simulink model "sm_radial_engine"  (R2021b)
settings: Solver=ode23t  StartTime=0.0  StopTime=10  RelTol=1e-3  EnableMultiTasking=on
model workspace (MATLAB code in the model file):
  | dgrey = [0.5 0.5 0.5];
  | lgrey = [0.7 0.7 0.7];
  | orange = [205 133 63]/255;
  | brown = [0.3 0.2 0.0];
  | lbrown = [139 90 43]/255;
  | yellow = [0.9 0.7 0.2];
  | 
  | rho_alum = 2700;
  | rho_steel = 8100;
  | 
  | Patm = 101100;
undefined symbols (not defined in the file): X, Y, Z
libraries: sm_lib x50, sm_radial_engine_lib x29, nesl_utility x2
(part 1 of 2)
Description:
  | Translational Interface : Radial Engine with Gas Force Model
  | 
  | This model simulates a five cylinder radial engine. The pressure dynamics inside the cylinders are modelled using the Simscape(TM) gas library. The 3D mechanical
  | components are modelled using Simscape Multibody(TM). See inside any of the blocks called "Force Model" to see how the 1D and 3D mechanical parts of the model are
  | interfaced. The pressure model is an ideal pressure source which applies pressure based on the crank angle. This model can be replaced with a more realistic pressure model
  | of the cylinder chamber. The cylinders fire in the sequence - A C E B D providing a power stroke every 144 deg of crank rotation.
settings Model: Creator=The MathWorks, Inc.  LastModifiedBy=The MathWorks, Inc.
settings SolverCC: AlgebraicLoopSolver=TrustRegion
settings DataIOCC: LimitDataPoints=on  SaveFormat=Array  SaveOutput=off  SignalLogging=off  SaveTime=off  ReturnWorkspaceOutputs=off  Refine=4
settings OptimizationCC: ExpressionDepthLimit=2147483647  LifeSpan=inf
settings DebuggingCC: ReadBeforeWriteMsg=DisableAll  WriteAfterWriteMsg=DisableAll  WriteAfterReadMsg=DisableAll  UnderspecifiedInitializationDetection=Classic  MergeDetectMultiDrivingBlocksExec=none  StateNameClashWarn=warning  SFUnexpectedBacktrackingDiag=warning  SFNoUnconditionalDefaultTransitionDiag=warning  SFExecutionAtInitializationDiag=none  SFMachineParentedDataDiag=warning  ArithmeticOperatorsInVariantConditions=warning
settings HardwareCC: ProdBitPerPointer=32  ProdBitPerSizeT=32  ProdBitPerPtrDiffT=32  ProdLargestAtomicFloat=None  ProdIntDivRoundTo=Undefined  ProdEndianess=Unspecified  ProdWordSize=32  ProdHWDeviceType=32-bit Generic
settings ModelReferenceCC: PropagateSignalLabelsOutOfModel=off
settings SFSimCC: SimUseLocalCustomCode=off  CustomCodeUndefinedFunction=UseInterfaceOnly
settings RTWCC: RTWUseLocalCustomCode=off
settings CodeAppCC: StateflowObjectComments=on
settings GRTTargetCC: TargetLangStandard=C89/C90 (ANSI)
settings ConfigComp: CovMetricSettings=dw  CovSaveCumulativeToWorkspaceVar=on  CovSaveSingleToWorkspaceVar=on  CovExternalEMLEnable=off
settings SimscapeCC: SimscapeNormalizeSystem=off  SimscapeNominalValues="[{\"value\":\"10\",\"unit\":\"V\"},{\"value\":\"1\",\"unit\":\"A\"},{\"value\":\"10\",\"unit\":\"N*m\"},{\"value\":\"10\",\"unit\":\"bar\"},{\"value\":\"100\",\"unit\":\"kJ/kg\"},{\"value\":\"1\",\"unit\":\"kW\"},{\"value\":\"300\",\"unit\":\"K\"},{\"value\":\"100\",\"unit\":\"cm^3/s\"},{\"value\":\"1\",\"unit\":\"kN\"},{\"value\":\"1\",\"unit\":\"g/cm^3\"},{\"value\":\"1\",\"unit\":\"l\"},{\"value\":\"1\",\"unit\":\"cm^2\"},{\"value\":\"60\",\"unit\":\"Hz\"}]"  SimscapeLogType=all  SimscapeLogSimulationStatistics=on  SimscapeLogName=simlog_sm_radial_engine  SimscapeLogLimitData=off
settings ConfigurationSet: Description=SimMechanics 2G
settings ExplorerConfigSet: InternalSimMechanicsExplorerSettings="<ExplorerConfiguration><canonicalview>default</canonicalview><AnimationSetting><BasePlaybackSpeed>1.0</BasePlaybackSpeed><PlaybackSpeedFactor>1.0</PlaybackSpeedFactor></AnimationSetting><TilePanel><TileInfo><Tiles Columns=\"1\" Count=\"1\" Rows=\"1\"><Column Left=\"2\" Weight=\"1\"/><Column Left=\"824\"/><Row Top=\"2\" Weight=\"1\"/><Row Top=\"666\"/><Tile Height=\"1\" Width=\"1\" X=\"0\" Y=\"0\"/></Tiles></TileInfo><SceneInfo><SceneViewer><BGColor><R>0.60000002384185791</R><G>0.60000002384185791</G><B>0.60000002384185791</B></BGColor><Camera><DoPerspective>off</DoPerspective><Position><X>1.3559688361863762</X><Y>-1.31712347590729295</Y><Z>1.392123463986364</Z></Position><Center><X>0.038845360279083252</X><Y>0</Y><Z>0.0749999880790710449</Z></Center><Up><X>-0.408248290463863073</X><Y>0.408248290463863073</Y><Z>0.816496580927726145</Z></Up><ViewLimDist>1</ViewLimDist><YLim>1.12278851172349969</YLim><XLim>1.3936290992842828</XLim></Camera></SceneViewer></SceneInfo></TilePanel><MechEditorPanel><Cameras/><GfxPanelCameraMap/><VideoCreator><PlaybackSpeedRatio>1.0</PlaybackSpeedRatio><FrameRate>30</FrameRate><VideoFormat>Motion JPEG AVI</VideoFormat><FrameSize>auto</FrameSize></VideoCreator></MechEditorPanel></ExplorerConfiguration>"

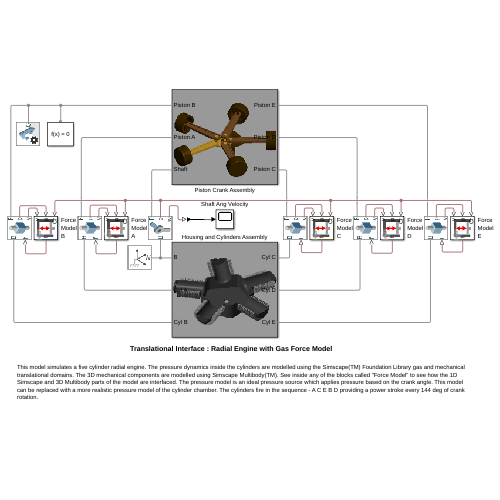
[thumbnail: Simulink's stored preview of the top-level diagram]
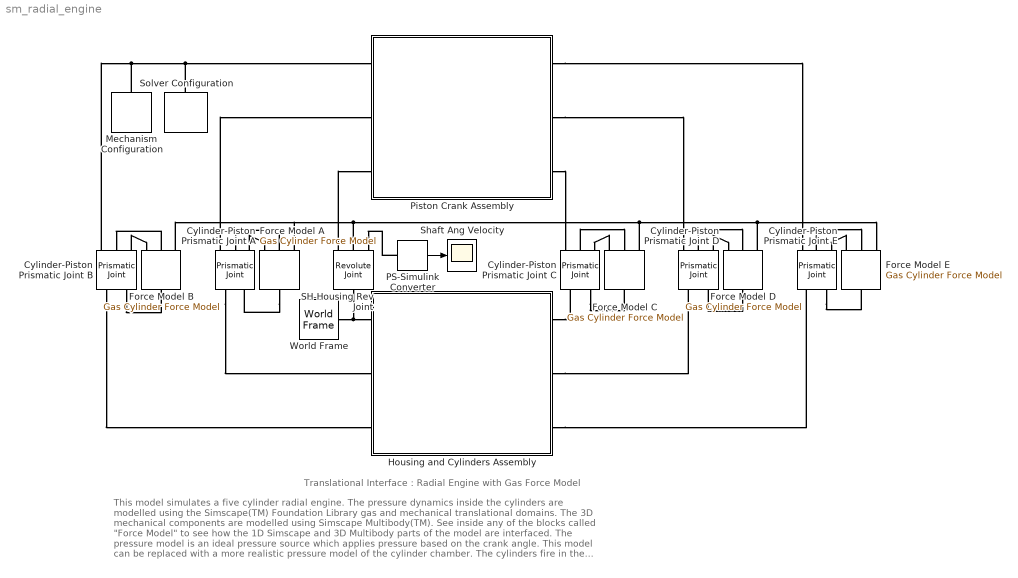
== system sm_radial_engine ==
  note: This model simulates a five cylinder radial engine. The pressure dynamics inside the cylinders are modelled using the Simscape(TM) Foundation Library gas and mechanical translational domains. The 3D mechanical components are modelled using Simscape Multibody(TM). See inside any of the blocks called "Force Model" to see how the 1D Simscape and 3D Multibody parts of the model are interfaced. The pressure model is an ideal pressure source which applies pressure based on the crank angle. This model can be replaced with a more realistic pressure model of the cylinder chamber. The cylinders fire in the sequence - A C E B D providing a power stroke every 144 deg of crank rotation.
  note: Translational Interface : Radial Engine with Gas Force Model
  Cylinder-Piston Prismatic Joint A : sm_lib/Joints/Prismatic Joint  JointMode=Normal  SenseConstraintForce=off  SenseConstraintForceX=off  SenseConstraintForceY=off  SenseConstraintForceZ=off  SenseConstraintTorque=off  SenseConstraintTorqueX=off  SenseConstraintTorqueY=off  SenseConstraintTorqueZ=off  SenseTotalForce=off  SenseTotalForceX=off  SenseTotalForceY=off  SenseTotalForceZ=off  SenseTotalTorque=off  SenseTotalTorqueX=off  SenseTotalTorqueY=off  SenseTotalTorqueZ=off  CompositeWrenchDir=FollowerOnBase  CompositeWrenchFrame=BaseFrame  EquilibriumPosition=0  EquilibriumPositionUnits=m  SpringStiffness=0  SpringStiffnessUnits=N/m  DampingCoefficient=0  DampingCoefficientUnits=N/(m/s)  TorqueActuationMode=InputTorque  MotionActuationMode=ComputedMotion  SensePosition=on  SenseVelocity=on  SenseAcceleration=off  SenseTorqueForce=off  SenseLowerLimitTorqueForce=off  SenseUpperLimitTorqueForce=off  LowerLimitSpecify=off  LowerLimitBound=-1  LowerLimitBoundUnits=m  LowerLimitStiffness=1e6  LowerLimitStiffnessUnits=N/m  LowerLimitDamping=1e3  LowerLimitDampingUnits=N/(m/s)  LowerLimitTransitionRegionWidth=1e-4  LowerLimitTransitionRegionWidthUnits=m  UpperLimitSpecify=off  UpperLimitBound=1  UpperLimitBoundUnits=m  UpperLimitStiffness=1e6  UpperLimitStiffnessUnits=N/m  UpperLimitDamping=1e3  UpperLimitDampingUnits=N/(m/s)  UpperLimitTransitionRegionWidth=1e-4  UpperLimitTransitionRegionWidthUnits=m  PositionTargetSpecify=on  PositionTargetPriority=Low  PositionTargetValue=-25  PositionTargetValueUnits=cm  VelocityTargetSpecify=off  VelocityTargetPriority=High  VelocityTargetValue=0  VelocityTargetValueUnits=m/s
  Cylinder-Piston Prismatic Joint B : sm_lib/Joints/Prismatic Joint  JointMode=Normal  SenseConstraintForce=off  SenseConstraintForceX=off  SenseConstraintForceY=off  SenseConstraintForceZ=off  SenseConstraintTorque=off  SenseConstraintTorqueX=off  SenseConstraintTorqueY=off  SenseConstraintTorqueZ=off  SenseTotalForce=off  SenseTotalForceX=off  SenseTotalForceY=off  SenseTotalForceZ=off  SenseTotalTorque=off  SenseTotalTorqueX=off  SenseTotalTorqueY=off  SenseTotalTorqueZ=off  CompositeWrenchDir=FollowerOnBase  CompositeWrenchFrame=BaseFrame  EquilibriumPosition=0  EquilibriumPositionUnits=m  SpringStiffness=0  SpringStiffnessUnits=N/m  DampingCoefficient=0  DampingCoefficientUnits=N/(m/s)  TorqueActuationMode=InputTorque  MotionActuationMode=ComputedMotion  SensePosition=on  SenseVelocity=on  SenseAcceleration=off  SenseTorqueForce=off  SenseLowerLimitTorqueForce=off  SenseUpperLimitTorqueForce=off  LowerLimitSpecify=off  LowerLimitBound=-1  LowerLimitBoundUnits=m  LowerLimitStiffness=1e6  LowerLimitStiffnessUnits=N/m  LowerLimitDamping=1e3  LowerLimitDampingUnits=N/(m/s)  LowerLimitTransitionRegionWidth=1e-4  LowerLimitTransitionRegionWidthUnits=m  UpperLimitSpecify=off  UpperLimitBound=1  UpperLimitBoundUnits=m  UpperLimitStiffness=1e6  UpperLimitStiffnessUnits=N/m  UpperLimitDamping=1e3  UpperLimitDampingUnits=N/(m/s)  UpperLimitTransitionRegionWidth=1e-4  UpperLimitTransitionRegionWidthUnits=m  PositionTargetSpecify=on  PositionTargetPriority=Low  PositionTargetValue=-25  PositionTargetValueUnits=cm  VelocityTargetSpecify=off  VelocityTargetPriority=High  VelocityTargetValue=0  VelocityTargetValueUnits=m/s
  Cylinder-Piston Prismatic Joint C : sm_lib/Joints/Prismatic Joint  JointMode=Normal  SenseConstraintForce=off  SenseConstraintForceX=off  SenseConstraintForceY=off  SenseConstraintForceZ=off  SenseConstraintTorque=off  SenseConstraintTorqueX=off  SenseConstraintTorqueY=off  SenseConstraintTorqueZ=off  SenseTotalForce=off  SenseTotalForceX=off  SenseTotalForceY=off  SenseTotalForceZ=off  SenseTotalTorque=off  SenseTotalTorqueX=off  SenseTotalTorqueY=off  SenseTotalTorqueZ=off  CompositeWrenchDir=FollowerOnBase  CompositeWrenchFrame=BaseFrame  EquilibriumPosition=0  EquilibriumPositionUnits=m  SpringStiffness=0  SpringStiffnessUnits=N/m  DampingCoefficient=0  DampingCoefficientUnits=N/(m/s)  TorqueActuationMode=InputTorque  MotionActuationMode=ComputedMotion  SensePosition=on  SenseVelocity=on  SenseAcceleration=off  SenseTorqueForce=off  SenseLowerLimitTorqueForce=off  SenseUpperLimitTorqueForce=off  LowerLimitSpecify=off  LowerLimitBound=-1  LowerLimitBoundUnits=m  LowerLimitStiffness=1e6  LowerLimitStiffnessUnits=N/m  LowerLimitDamping=1e3  LowerLimitDampingUnits=N/(m/s)  LowerLimitTransitionRegionWidth=1e-4  LowerLimitTransitionRegionWidthUnits=m  UpperLimitSpecify=off  UpperLimitBound=1  UpperLimitBoundUnits=m  UpperLimitStiffness=1e6  UpperLimitStiffnessUnits=N/m  UpperLimitDamping=1e3  UpperLimitDampingUnits=N/(m/s)  UpperLimitTransitionRegionWidth=1e-4  UpperLimitTransitionRegionWidthUnits=m  PositionTargetSpecify=on  PositionTargetPriority=Low  PositionTargetValue=-25  PositionTargetValueUnits=cm  VelocityTargetSpecify=off  VelocityTargetPriority=High  VelocityTargetValue=0  VelocityTargetValueUnits=m/s
  Cylinder-Piston Prismatic Joint D : sm_lib/Joints/Prismatic Joint  JointMode=Normal  SenseConstraintForce=off  SenseConstraintForceX=off  SenseConstraintForceY=off  SenseConstraintForceZ=off  SenseConstraintTorque=off  SenseConstraintTorqueX=off  SenseConstraintTorqueY=off  SenseConstraintTorqueZ=off  SenseTotalForce=off  SenseTotalForceX=off  SenseTotalForceY=off  SenseTotalForceZ=off  SenseTotalTorque=off  SenseTotalTorqueX=off  SenseTotalTorqueY=off  SenseTotalTorqueZ=off  CompositeWrenchDir=FollowerOnBase  CompositeWrenchFrame=BaseFrame  EquilibriumPosition=0  EquilibriumPositionUnits=m  SpringStiffness=0  SpringStiffnessUnits=N/m  DampingCoefficient=0  DampingCoefficientUnits=N/(m/s)  TorqueActuationMode=InputTorque  MotionActuationMode=ComputedMotion  SensePosition=on  SenseVelocity=on  SenseAcceleration=off  SenseTorqueForce=off  SenseLowerLimitTorqueForce=off  SenseUpperLimitTorqueForce=off  LowerLimitSpecify=off  LowerLimitBound=-1  LowerLimitBoundUnits=m  LowerLimitStiffness=1e6  LowerLimitStiffnessUnits=N/m  LowerLimitDamping=1e3  LowerLimitDampingUnits=N/(m/s)  LowerLimitTransitionRegionWidth=1e-4  LowerLimitTransitionRegionWidthUnits=m  UpperLimitSpecify=off  UpperLimitBound=1  UpperLimitBoundUnits=m  UpperLimitStiffness=1e6  UpperLimitStiffnessUnits=N/m  UpperLimitDamping=1e3  UpperLimitDampingUnits=N/(m/s)  UpperLimitTransitionRegionWidth=1e-4  UpperLimitTransitionRegionWidthUnits=m  PositionTargetSpecify=on  PositionTargetPriority=Low  PositionTargetValue=-25  PositionTargetValueUnits=cm  VelocityTargetSpecify=off  VelocityTargetPriority=High  VelocityTargetValue=0  VelocityTargetValueUnits=m/s
  Cylinder-Piston Prismatic Joint E : sm_lib/Joints/Prismatic Joint  JointMode=Normal  SenseConstraintForce=off  SenseConstraintForceX=off  SenseConstraintForceY=off  SenseConstraintForceZ=off  SenseConstraintTorque=off  SenseConstraintTorqueX=off  SenseConstraintTorqueY=off  SenseConstraintTorqueZ=off  SenseTotalForce=off  SenseTotalForceX=off  SenseTotalForceY=off  SenseTotalForceZ=off  SenseTotalTorque=off  SenseTotalTorqueX=off  SenseTotalTorqueY=off  SenseTotalTorqueZ=off  CompositeWrenchDir=FollowerOnBase  CompositeWrenchFrame=BaseFrame  EquilibriumPosition=0  EquilibriumPositionUnits=m  SpringStiffness=0  SpringStiffnessUnits=N/m  DampingCoefficient=0  DampingCoefficientUnits=N/(m/s)  TorqueActuationMode=InputTorque  MotionActuationMode=ComputedMotion  SensePosition=on  SenseVelocity=on  SenseAcceleration=off  SenseTorqueForce=off  SenseLowerLimitTorqueForce=off  SenseUpperLimitTorqueForce=off  LowerLimitSpecify=off  LowerLimitBound=-1  LowerLimitBoundUnits=m  LowerLimitStiffness=1e6  LowerLimitStiffnessUnits=N/m  LowerLimitDamping=1e3  LowerLimitDampingUnits=N/(m/s)  LowerLimitTransitionRegionWidth=1e-4  LowerLimitTransitionRegionWidthUnits=m  UpperLimitSpecify=off  UpperLimitBound=1  UpperLimitBoundUnits=m  UpperLimitStiffness=1e6  UpperLimitStiffnessUnits=N/m  UpperLimitDamping=1e3  UpperLimitDampingUnits=N/(m/s)  UpperLimitTransitionRegionWidth=1e-4  UpperLimitTransitionRegionWidthUnits=m  PositionTargetSpecify=on  PositionTargetPriority=Low  PositionTargetValue=-25  PositionTargetValueUnits=cm  VelocityTargetSpecify=off  VelocityTargetPriority=High  VelocityTargetValue=0  VelocityTargetValueUnits=m/s
  Force Model A : sm_radial_engine_lib/Gas Cylinder Force Model  PA=pi*169  Lc=50  Patm=Patm  Ppk=20000  Pi=20230  sta=-10  pka=10  ena=80
      settings: SourceProductBaseCode=MS
  Force Model B : sm_radial_engine_lib/Gas Cylinder Force Model  PA=pi*169  Lc=50  Patm=Patm  Ppk=20000  Pi=0  sta=422  pka=442  ena=522
      settings: SourceProductBaseCode=MS
  Force Model C : sm_radial_engine_lib/Gas Cylinder Force Model  PA=pi*169  Lc=50  Patm=Patm  Ppk=20000  Pi=0  sta=134  pka=154  ena=234
      settings: SourceProductBaseCode=MS
  Force Model D : sm_radial_engine_lib/Gas Cylinder Force Model  PA=pi*169  Lc=50  Patm=Patm  Ppk=20000  Pi=0  sta=566  pka=586  ena=666
      settings: SourceProductBaseCode=MS
  Force Model E : sm_radial_engine_lib/Gas Cylinder Force Model  PA=pi*169  Lc=50  Patm=Patm  Ppk=20000  Pi=0  sta=278  pka=298  ena=378
      settings: SourceProductBaseCode=MS
  Housing and Cylinders Assembly : Subsystem
      mask Display:
      | image('sm_radial_engine_housecyl.png');
      | port_label('RConn',1,'Cyl C');
      | port_label('RConn',2,'Cyl D');
      | port_label('RConn',3,'Cyl E');
      | port_label('LConn',1,'B');
      | port_label('LConn',2,'Cyl A');
      | port_label('LConn',3,'Cyl B');
  Mechanism Configuration : sm_lib/Utilities/Mechanism Configuration  UniformGravity=Constant  GravityVector=[0 0 -9.81]  GravityUnits=m/s^2  LinearizationDelta=0.001  JointModeTransitionNonlinearIterations=2
  PS-Simulink Converter : nesl_utility/PS-Simulink Converter  PhysicalDomain=network_engine_domain  SubClassName=ps_output  LeftPortType=input  RightPortType=output  PseudoPeriodic=off  Frequencies=[]  Unit=rpm  AffineConversion=off
      settings: SourceProductBaseCode=PW,SS
  Piston Crank Assembly : Subsystem
      mask Display:
      | image('sm_radial_engine_crankpis.png');
      | port_label('RConn',1,'Piston E');
      | port_label('RConn',2,'Piston D');
      | port_label('RConn',3,'Piston C');
      | port_label('LConn',1,'Piston B');
      | port_label('LConn',2,'Piston A');
      | port_label('LConn',3,'Shaft');
  SH-Housing Rev Joint : sm_lib/Joints/Revolute Joint  JointMode=Normal  SenseConstraintForce=off  SenseConstraintForceX=off  SenseConstraintForceY=off  SenseConstraintForceZ=off  SenseConstraintTorque=off  SenseConstraintTorqueX=off  SenseConstraintTorqueY=off  SenseConstraintTorqueZ=off  SenseTotalForce=off  SenseTotalForceX=off  SenseTotalForceY=off  SenseTotalForceZ=off  SenseTotalTorque=off  SenseTotalTorqueX=off  SenseTotalTorqueY=off  SenseTotalTorqueZ=off  CompositeWrenchDir=FollowerOnBase  CompositeWrenchFrame=BaseFrame  EquilibriumPosition=0  EquilibriumPositionUnits=deg  SpringStiffness=0  SpringStiffnessUnits=N*m/deg  DampingCoefficient=0.05  DampingCoefficientUnits=N*m/(deg/s)  TorqueActuationMode=NoTorque  MotionActuationMode=ComputedMotion  SensePosition=on  SenseVelocity=on  SenseAcceleration=off  SenseTorqueForce=off  SenseLowerLimitTorqueForce=off  SenseUpperLimitTorqueForce=off  LowerLimitSpecify=off  LowerLimitBound=-90  LowerLimitBoundUnits=deg  LowerLimitStiffness=1e4  LowerLimitStiffnessUnits=N*m/deg  LowerLimitDamping=10  LowerLimitDampingUnits=N*m/(deg/s)  LowerLimitTransitionRegionWidth=0.1  LowerLimitTransitionRegionWidthUnits=deg  UpperLimitSpecify=off  UpperLimitBound=90  UpperLimitBoundUnits=deg  UpperLimitStiffness=1e4  UpperLimitStiffnessUnits=N*m/deg  UpperLimitDamping=10  UpperLimitDampingUnits=N*m/(deg/s)  UpperLimitTransitionRegionWidth=0.1  UpperLimitTransitionRegionWidthUnits=deg  PositionTargetSpecify=on  PositionTargetPriority=High  PositionTargetValue=10  PositionTargetValueUnits=deg  VelocityTargetSpecify=off  VelocityTargetPriority=High  VelocityTargetValue=0  VelocityTargetValueUnits=deg/s
  Shaft Ang Velocity : Scope
  Solver Configuration : nesl_utility/Solver Configuration  PhysicalDomain=network_engine_domain  SubClassName=solver  LeftPortType=input  RightPortType=generic  Tones=[]  Harmonics=[]  SimulateNoise=off  Profile=off  UseLocalSampling=off  EnableSwitchedLinearOptims=on  FrequencyDomain=off  UseCCode=off  RelTol=0.001  AbsTol=1e-06  MinStep=1e-09  ToWorkspace=off  RevertToSquareIcSolve=off  NumHomotopyIterations=100  PhasorMode=off  PhasorModeNumHarmonics=1  DoDC=off  ResidualTolerance=1e-9  UseLocalSolver=off  LocalSolverChoice=NE_BACKWARD_EULER_ADVANCER  LocalSolverSampleTime=.01  DoFixedCost=off  MaxNonlinIter=3  MaxModeIter=2  ComputeImpulses=off  ImpulseIterations=2  LinearAlgebra=Sparse  EquationFormulation=NE_TIME_EF  DelaysMemoryBudget=1024  AutomaticFiltering=on  FilteringTimeConstant=0.001  PartitionStorageMethod=AS_NEEDED  PartitionMemoryBudget=1024  PartitionMethod=FAST
      settings: SourceProductBaseCode=PW,SS
  World Frame : sm_lib/Frames and Transforms/World Frame
  wires:
  PS-Simulink Converter/1 -> Shaft Ang Velocity/1
  connections:
  Cylinder-Piston Prismatic Joint C/LConn2 -- Force Model C/LConn1
  Cylinder-Piston Prismatic Joint E/LConn2 -- Force Model E/LConn1
  Force Model D/LConn1 -- Cylinder-Piston Prismatic Joint D/LConn2
  Cylinder-Piston Prismatic Joint B/LConn2 -- Force Model B/LConn1
  Cylinder-Piston Prismatic Joint B/RConn1 -- Piston Crank Assembly/LConn1 -- Solver Configuration/RConn1 -- Mechanism Configuration/RConn1
  Cylinder-Piston Prismatic Joint B/LConn1 -- Housing and Cylinders Assembly/LConn3
  Force Model A/LConn1 -- Cylinder-Piston Prismatic Joint A/LConn2
  Cylinder-Piston Prismatic Joint A/RConn1 -- Piston Crank Assembly/LConn2
  Cylinder-Piston Prismatic Joint A/LConn1 -- Housing and Cylinders Assembly/LConn2
  Piston Crank Assembly/RConn1 -- Cylinder-Piston Prismatic Joint E/RConn1
  Housing and Cylinders Assembly/RConn3 -- Cylinder-Piston Prismatic Joint E/LConn1
  Piston Crank Assembly/RConn2 -- Cylinder-Piston Prismatic Joint D/RConn1
  Housing and Cylinders Assembly/RConn2 -- Cylinder-Piston Prismatic Joint D/LConn1
  Piston Crank Assembly/RConn3 -- Cylinder-Piston Prismatic Joint C/RConn1
  Housing and Cylinders Assembly/RConn1 -- Cylinder-Piston Prismatic Joint C/LConn1
  SH-Housing Rev Joint/RConn1 -- Piston Crank Assembly/LConn3
  SH-Housing Rev Joint/LConn1 -- Housing and Cylinders Assembly/LConn1 -- World Frame/RConn1
  SH-Housing Rev Joint/RConn2 -- Force Model A/RConn3 -- Force Model B/RConn3 -- Force Model C/RConn3 -- Force Model E/RConn3 -- Force Model D/RConn3
  PS-Simulink Converter/LConn1 -- SH-Housing Rev Joint/RConn3
  Cylinder-Piston Prismatic Joint B/RConn3 -- Force Model B/RConn1
  Cylinder-Piston Prismatic Joint A/RConn3 -- Force Model A/RConn1
  Force Model A/RConn2 -- Cylinder-Piston Prismatic Joint A/RConn2
  Force Model B/RConn2 -- Cylinder-Piston Prismatic Joint B/RConn2
  Force Model C/RConn1 -- Cylinder-Piston Prismatic Joint C/RConn3
  Cylinder-Piston Prismatic Joint C/RConn2 -- Force Model C/RConn2
  Cylinder-Piston Prismatic Joint D/RConn3 -- Force Model D/RConn1
  Cylinder-Piston Prismatic Joint D/RConn2 -- Force Model D/RConn2
  Force Model E/RConn1 -- Cylinder-Piston Prismatic Joint E/RConn3
  Cylinder-Piston Prismatic Joint E/RConn2 -- Force Model E/RConn2

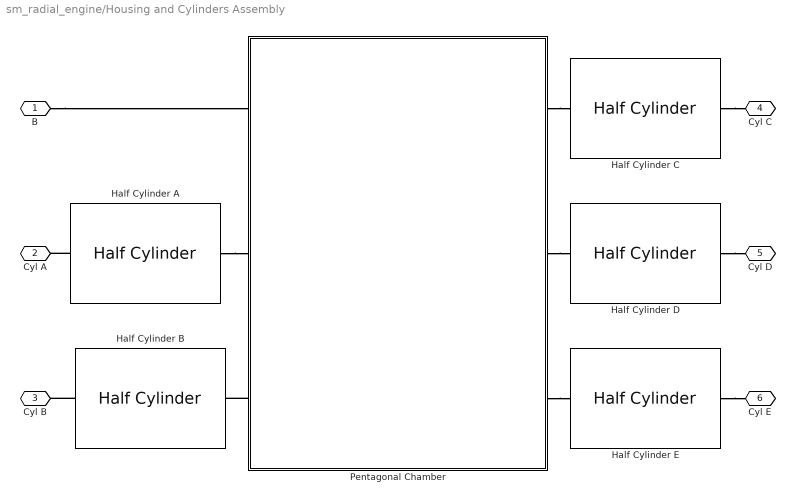
== system sm_radial_engine/Housing and Cylinders Assembly ==
  Half Cylinder A : sm_radial_engine_lib/Half Cylinder  L=50  Ro=15  Ri=13  Rf=20  Tf=10  Sf=30  Rv=2  cclr=[0.3 0.3 0.3]  fclr=[0.7 0.7 0.7]  rho=2700
      settings: SourceProductBaseCode=MS
  Half Cylinder B : sm_radial_engine_lib/Half Cylinder  L=50  Ro=15  Ri=13  Rf=20  Tf=10  Sf=30  Rv=2  cclr=[0.3 0.3 0.3]  fclr=[0.7 0.7 0.7]  rho=2700
      settings: SourceProductBaseCode=MS
  Half Cylinder C : sm_radial_engine_lib/Half Cylinder  L=50  Ro=15  Ri=13  Rf=20  Tf=10  Sf=30  Rv=2  cclr=[0.3 0.3 0.3]  fclr=[0.7 0.7 0.7]  rho=2700
      settings: SourceProductBaseCode=MS
  Half Cylinder D : sm_radial_engine_lib/Half Cylinder  L=50  Ro=15  Ri=13  Rf=20  Tf=10  Sf=30  Rv=2  cclr=[0.3 0.3 0.3]  fclr=[0.7 0.7 0.7]  rho=2700
      settings: SourceProductBaseCode=MS
  Half Cylinder E : sm_radial_engine_lib/Half Cylinder  L=50  Ro=15  Ri=13  Rf=20  Tf=10  Sf=30  Rv=2  cclr=[0.3 0.3 0.3]  fclr=[0.7 0.7 0.7]  rho=2700
      settings: SourceProductBaseCode=MS
  Pentagonal Chamber : Subsystem  mask(Pentagonal Chamber){Rc=40, Lw=45, Tw=2, Hw=25, Rs=5, Rm=17.0, clr=[0.3 0.3 0.3], rho=2700}
      mask prompts: Rc "Circumcircle radius (cm)"; Lw "Wall straight section length (cm)"; Tw "Wall thickness (cm)"; Hw "Wall height (cm)"; Rs "Shaft hole radius (cm):"; Rm "Mounting hole radius (cm)"; clr "Color [r g b]:"; rho "Density (kg/m^3):"
      mask help: This block models the pentagonal chamber that houses the five cylinders, drive shaft, fly wheel, cranks and pistons.
      mask init:
      | d36 = 36*pi/180;
      | 
      | % Curved wall radius
      | Rcw = Rc-(Lw/2)/tan(d36);
      | 
      | % Curved wall distance from center
      | Dcw = Rcw + (Lw/2)/sin(d36);
      | 
      | % Base cross section
      | theta = linspace(-d36,d36,72)';
      | arc = [Rcw*cos(theta)+(Dcw-Rcw+Tw/2) Rcw*sin(theta)];
      | base_xsec = [];
      | for idx=36:72:324
      |     th = idx*pi/180;
      |     RotzT = [cos(th) sin(th); -sin(th) cos(th)];
      |     base_xsec = [base_xsec; arc*RotzT];
      | end
      | 
      | base_xsec(end,1:2) = base_xsec(1,1:2);
      | 
      | % Hole
      | theta = linspace(0,-2*pi,200)';
      | base_xsec = [base_xsec; Rs*cos(theta) Rs*sin(theta)];
      mask DialogControl ParameterTabVar0 Prompt: Dimensions
      mask DialogControl ParameterTabVar01 Prompt: Material Properties
      mask Display:
      | image('sm_radial_engine_pcham.png');
      | port_label('LConn',1,'B');
      | port_label('LConn',2,'MA');
      | port_label('LConn',3,'MB');
      | port_label('RConn',1,'MC');
      | port_label('RConn',2,'MD');
      | port_label('RConn',3,'ME');
  B : PMIOPort  Side=Left
  Cyl A : PMIOPort  Port=2  Side=Left
  Cyl B : PMIOPort  Port=3  Side=Left
  Cyl C : PMIOPort  Port=4  Side=Right
  Cyl D : PMIOPort  Port=5  Side=Right
  Cyl E : PMIOPort  Port=6  Side=Right
  connections:
  Pentagonal Chamber/RConn3 -- Half Cylinder E/LConn1
  Half Cylinder C/RConn1 -- Cyl C/RConn1
  Half Cylinder E/RConn1 -- Cyl E/RConn1
  Pentagonal Chamber/RConn2 -- Half Cylinder D/LConn1
  Pentagonal Chamber/RConn1 -- Half Cylinder C/LConn1
  Half Cylinder D/RConn1 -- Cyl D/RConn1
  Half Cylinder A/RConn1 -- Cyl A/RConn1
  Pentagonal Chamber/LConn3 -- Half Cylinder B/LConn1
  Half Cylinder B/RConn1 -- Cyl B/RConn1
  B/RConn1 -- Pentagonal Chamber/LConn1
  Half Cylinder A/LConn1 -- Pentagonal Chamber/LConn2

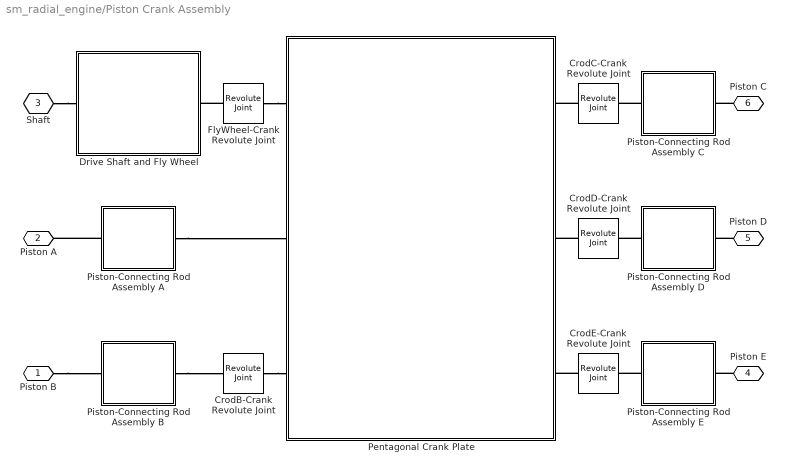
== system sm_radial_engine/Piston Crank Assembly ==
  "CrodB-Crank Revolute Joint " : sm_lib/Joints/Revolute Joint  JointMode=Normal  SenseConstraintForce=off  SenseConstraintForceX=off  SenseConstraintForceY=off  SenseConstraintForceZ=off  SenseConstraintTorque=off  SenseConstraintTorqueX=off  SenseConstraintTorqueY=off  SenseConstraintTorqueZ=off  SenseTotalForce=off  SenseTotalForceX=off  SenseTotalForceY=off  SenseTotalForceZ=off  SenseTotalTorque=off  SenseTotalTorqueX=off  SenseTotalTorqueY=off  SenseTotalTorqueZ=off  CompositeWrenchDir=FollowerOnBase  CompositeWrenchFrame=BaseFrame  EquilibriumPosition=0  EquilibriumPositionUnits=deg  SpringStiffness=0  SpringStiffnessUnits=N*m/deg  DampingCoefficient=0  DampingCoefficientUnits=N*m/(deg/s)  TorqueActuationMode=NoTorque  MotionActuationMode=ComputedMotion  SensePosition=off  SenseVelocity=off  SenseAcceleration=off  SenseTorqueForce=off  SenseLowerLimitTorqueForce=off  SenseUpperLimitTorqueForce=off  LowerLimitSpecify=off  LowerLimitBound=-90  LowerLimitBoundUnits=deg  LowerLimitStiffness=1e4  LowerLimitStiffnessUnits=N*m/deg  LowerLimitDamping=10  LowerLimitDampingUnits=N*m/(deg/s)  LowerLimitTransitionRegionWidth=0.1  LowerLimitTransitionRegionWidthUnits=deg  UpperLimitSpecify=off  UpperLimitBound=90  UpperLimitBoundUnits=deg  UpperLimitStiffness=1e4  UpperLimitStiffnessUnits=N*m/deg  UpperLimitDamping=10  UpperLimitDampingUnits=N*m/(deg/s)  UpperLimitTransitionRegionWidth=0.1  UpperLimitTransitionRegionWidthUnits=deg  PositionTargetSpecify=off  PositionTargetPriority=Low  PositionTargetValue=0  PositionTargetValueUnits=deg  VelocityTargetSpecify=off  VelocityTargetPriority=High  VelocityTargetValue=0  VelocityTargetValueUnits=deg/s
  "CrodC-Crank Revolute Joint " : sm_lib/Joints/Revolute Joint  JointMode=Normal  SenseConstraintForce=off  SenseConstraintForceX=off  SenseConstraintForceY=off  SenseConstraintForceZ=off  SenseConstraintTorque=off  SenseConstraintTorqueX=off  SenseConstraintTorqueY=off  SenseConstraintTorqueZ=off  SenseTotalForce=off  SenseTotalForceX=off  SenseTotalForceY=off  SenseTotalForceZ=off  SenseTotalTorque=off  SenseTotalTorqueX=off  SenseTotalTorqueY=off  SenseTotalTorqueZ=off  CompositeWrenchDir=FollowerOnBase  CompositeWrenchFrame=BaseFrame  EquilibriumPosition=0  EquilibriumPositionUnits=deg  SpringStiffness=0  SpringStiffnessUnits=N*m/deg  DampingCoefficient=0  DampingCoefficientUnits=N*m/(deg/s)  TorqueActuationMode=NoTorque  MotionActuationMode=ComputedMotion  SensePosition=off  SenseVelocity=off  SenseAcceleration=off  SenseTorqueForce=off  SenseLowerLimitTorqueForce=off  SenseUpperLimitTorqueForce=off  LowerLimitSpecify=off  LowerLimitBound=-90  LowerLimitBoundUnits=deg  LowerLimitStiffness=1e4  LowerLimitStiffnessUnits=N*m/deg  LowerLimitDamping=10  LowerLimitDampingUnits=N*m/(deg/s)  LowerLimitTransitionRegionWidth=0.1  LowerLimitTransitionRegionWidthUnits=deg  UpperLimitSpecify=off  UpperLimitBound=90  UpperLimitBoundUnits=deg  UpperLimitStiffness=1e4  UpperLimitStiffnessUnits=N*m/deg  UpperLimitDamping=10  UpperLimitDampingUnits=N*m/(deg/s)  UpperLimitTransitionRegionWidth=0.1  UpperLimitTransitionRegionWidthUnits=deg  PositionTargetSpecify=off  PositionTargetPriority=Low  PositionTargetValue=180  PositionTargetValueUnits=deg  VelocityTargetSpecify=off  VelocityTargetPriority=High  VelocityTargetValue=0  VelocityTargetValueUnits=deg/s
  "CrodD-Crank Revolute Joint " : sm_lib/Joints/Revolute Joint  JointMode=Normal  SenseConstraintForce=off  SenseConstraintForceX=off  SenseConstraintForceY=off  SenseConstraintForceZ=off  SenseConstraintTorque=off  SenseConstraintTorqueX=off  SenseConstraintTorqueY=off  SenseConstraintTorqueZ=off  SenseTotalForce=off  SenseTotalForceX=off  SenseTotalForceY=off  SenseTotalForceZ=off  SenseTotalTorque=off  SenseTotalTorqueX=off  SenseTotalTorqueY=off  SenseTotalTorqueZ=off  CompositeWrenchDir=FollowerOnBase  CompositeWrenchFrame=BaseFrame  EquilibriumPosition=0  EquilibriumPositionUnits=deg  SpringStiffness=0  SpringStiffnessUnits=N*m/deg  DampingCoefficient=0  DampingCoefficientUnits=N*m/(deg/s)  TorqueActuationMode=NoTorque  MotionActuationMode=ComputedMotion  SensePosition=off  SenseVelocity=off  SenseAcceleration=off  SenseTorqueForce=off  SenseLowerLimitTorqueForce=off  SenseUpperLimitTorqueForce=off  LowerLimitSpecify=off  LowerLimitBound=-90  LowerLimitBoundUnits=deg  LowerLimitStiffness=1e4  LowerLimitStiffnessUnits=N*m/deg  LowerLimitDamping=10  LowerLimitDampingUnits=N*m/(deg/s)  LowerLimitTransitionRegionWidth=0.1  LowerLimitTransitionRegionWidthUnits=deg  UpperLimitSpecify=off  UpperLimitBound=90  UpperLimitBoundUnits=deg  UpperLimitStiffness=1e4  UpperLimitStiffnessUnits=N*m/deg  UpperLimitDamping=10  UpperLimitDampingUnits=N*m/(deg/s)  UpperLimitTransitionRegionWidth=0.1  UpperLimitTransitionRegionWidthUnits=deg  PositionTargetSpecify=off  PositionTargetPriority=Low  PositionTargetValue=180  PositionTargetValueUnits=deg  VelocityTargetSpecify=off  VelocityTargetPriority=High  VelocityTargetValue=0  VelocityTargetValueUnits=deg/s
  "CrodE-Crank Revolute Joint " : sm_lib/Joints/Revolute Joint  JointMode=Normal  SenseConstraintForce=off  SenseConstraintForceX=off  SenseConstraintForceY=off  SenseConstraintForceZ=off  SenseConstraintTorque=off  SenseConstraintTorqueX=off  SenseConstraintTorqueY=off  SenseConstraintTorqueZ=off  SenseTotalForce=off  SenseTotalForceX=off  SenseTotalForceY=off  SenseTotalForceZ=off  SenseTotalTorque=off  SenseTotalTorqueX=off  SenseTotalTorqueY=off  SenseTotalTorqueZ=off  CompositeWrenchDir=FollowerOnBase  CompositeWrenchFrame=BaseFrame  EquilibriumPosition=0  EquilibriumPositionUnits=deg  SpringStiffness=0  SpringStiffnessUnits=N*m/deg  DampingCoefficient=0  DampingCoefficientUnits=N*m/(deg/s)  TorqueActuationMode=NoTorque  MotionActuationMode=ComputedMotion  SensePosition=off  SenseVelocity=off  SenseAcceleration=off  SenseTorqueForce=off  SenseLowerLimitTorqueForce=off  SenseUpperLimitTorqueForce=off  LowerLimitSpecify=off  LowerLimitBound=-90  LowerLimitBoundUnits=deg  LowerLimitStiffness=1e4  LowerLimitStiffnessUnits=N*m/deg  LowerLimitDamping=10  LowerLimitDampingUnits=N*m/(deg/s)  LowerLimitTransitionRegionWidth=0.1  LowerLimitTransitionRegionWidthUnits=deg  UpperLimitSpecify=off  UpperLimitBound=90  UpperLimitBoundUnits=deg  UpperLimitStiffness=1e4  UpperLimitStiffnessUnits=N*m/deg  UpperLimitDamping=10  UpperLimitDampingUnits=N*m/(deg/s)  UpperLimitTransitionRegionWidth=0.1  UpperLimitTransitionRegionWidthUnits=deg  PositionTargetSpecify=off  PositionTargetPriority=Low  PositionTargetValue=180  PositionTargetValueUnits=deg  VelocityTargetSpecify=off  VelocityTargetPriority=High  VelocityTargetValue=0  VelocityTargetValueUnits=deg/s
  Drive Shaft and Fly Wheel : Subsystem  mask(Drive Shaft and Fly Wheel){Rs=2, Ls=40, Rw=35, Tw=6, Rp=2, Lp=3.5, Dp=15, Ob=4, clr=brown, rho=rho_steel}
      mask prompts: Rs "Shaft radius (cm):"; Ls "Shaft length (cm):"; Rw "Flywheel radius (cm):"; Tw "Flywheel thickness(cm):"; Rp "Crank pin radius (cm):"; Lp "Crank pin length (cm):"; Dp "Crank pin distance (cm):"; Ob "Bearing offset (cm):"; clr "Color [r g b]:"; rho "Density (kg/m^3):"
      mask help: This block models a drive shaft and a rigidly attached fly wheel. The fly wheel has a hole which houses the crank plate pin. The port S corresponds to the shaft frame and the port CP corresponds to the hole frame.
      mask init:
      | % Fly Wheel
      | theta = [linspace(0,3*pi/4,100)'; linspace(5*pi/4,2*pi,100)'];
      | theta_ = linspace(2*pi,0,200)';
      | 
      | flywh_xsec = [Rw*cos(theta) Rw*sin(theta)];
      |           
      | shaft_xsec = [Rs*cos(theta) Rs*sin(theta)];
      mask Display:
      | image('sm_radial_engine_sfly.png');
      | port_label('RConn',1,'CP');
      | port_label('LConn',1,'S');
  FlyWheel-Crank Revolute Joint : sm_lib/Joints/Revolute Joint  JointMode=Normal  SenseConstraintForce=off  SenseConstraintForceX=off  SenseConstraintForceY=off  SenseConstraintForceZ=off  SenseConstraintTorque=off  SenseConstraintTorqueX=off  SenseConstraintTorqueY=off  SenseConstraintTorqueZ=off  SenseTotalForce=off  SenseTotalForceX=off  SenseTotalForceY=off  SenseTotalForceZ=off  SenseTotalTorque=off  SenseTotalTorqueX=off  SenseTotalTorqueY=off  SenseTotalTorqueZ=off  CompositeWrenchDir=FollowerOnBase  CompositeWrenchFrame=BaseFrame  EquilibriumPosition=0  EquilibriumPositionUnits=deg  SpringStiffness=0  SpringStiffnessUnits=N*m/deg  DampingCoefficient=0  DampingCoefficientUnits=N*m/(deg/s)  TorqueActuationMode=NoTorque  MotionActuationMode=ComputedMotion  SensePosition=off  SenseVelocity=off  SenseAcceleration=off  SenseTorqueForce=off  SenseLowerLimitTorqueForce=off  SenseUpperLimitTorqueForce=off  LowerLimitSpecify=off  LowerLimitBound=-90  LowerLimitBoundUnits=deg  LowerLimitStiffness=1e4  LowerLimitStiffnessUnits=N*m/deg  LowerLimitDamping=10  LowerLimitDampingUnits=N*m/(deg/s)  LowerLimitTransitionRegionWidth=0.1  LowerLimitTransitionRegionWidthUnits=deg  UpperLimitSpecify=off  UpperLimitBound=90  UpperLimitBoundUnits=deg  UpperLimitStiffness=1e4  UpperLimitStiffnessUnits=N*m/deg  UpperLimitDamping=10  UpperLimitDampingUnits=N*m/(deg/s)  UpperLimitTransitionRegionWidth=0.1  UpperLimitTransitionRegionWidthUnits=deg  PositionTargetSpecify=on  PositionTargetPriority=Low  PositionTargetValue=10  PositionTargetValueUnits=deg  VelocityTargetSpecify=off  VelocityTargetPriority=High  VelocityTargetValue=0  VelocityTargetValueUnits=deg/s
  Pentagonal Crank Plate : Subsystem  mask(Pentagonal Crank Plate){Rc=15, Rcp=2, Rp=2, Lp=3, Dp=10, T=1.5, clr=yellow, rho=rho_alum}
      mask prompts: Rc "Circumcircle radius (cm):"; Rcp "Crank pin hole radius (cm):"; Rp "Conn rod pin radius (cm):"; Lp "Conn rod pin length (cm):"; Dp "Conn rod pin distance (cm):"; T "Plate thickness (cm):"; clr "Color [r g b]:"; rho "Density (kg/m^3):"
      mask help: This block models a pentagonal plate with 4 pins for 4 connecting rods and another pin for the fly wheel. The five ports A-E correspond to the five frames where the connecting rods attach to the crank plate. The port SP corresponds to the pin frame that connects to the fly wheel.
      mask Display:
      | image('sm_radial_engine_cplate.png');
      | port_label('LConn',1,'SP');
      | port_label('LConn',2,'A');
      | port_label('LConn',3,'B');
      | port_label('RConn',1,'C');
      | port_label('RConn',2,'D');
      | port_label('RConn',3,'E');
  Piston-Connecting Rod Assembly A : Subsystem
  Piston-Connecting Rod Assembly B : Subsystem
  Piston-Connecting Rod Assembly C : Subsystem
  Piston-Connecting Rod Assembly D : Subsystem
  Piston-Connecting Rod Assembly E : Subsystem
  Piston B : PMIOPort  Side=Left
  Piston A : PMIOPort  Port=2  Side=Left
  Shaft : PMIOPort  Port=3  Side=Left
  Piston E : PMIOPort  Port=4  Side=Right
  Piston D : PMIOPort  Port=5  Side=Right
  Piston C : PMIOPort  Port=6  Side=Right
  connections:
  FlyWheel-Crank Revolute Joint/RConn1 -- Drive Shaft and Fly Wheel/RConn1
  "CrodD-Crank Revolute Joint "/RConn1 -- Pentagonal Crank Plate/RConn2
  FlyWheel-Crank Revolute Joint/LConn1 -- Pentagonal Crank Plate/LConn1
  Piston-Connecting Rod Assembly D/RConn1 -- "CrodD-Crank Revolute Joint "/LConn1
  Piston-Connecting Rod Assembly A/LConn1 -- Piston A/RConn1
  Piston E/RConn1 -- Piston-Connecting Rod Assembly E/LConn1
  "CrodC-Crank Revolute Joint "/RConn1 -- Pentagonal Crank Plate/RConn1
  Piston-Connecting Rod Assembly A/RConn1 -- Pentagonal Crank Plate/LConn2
  Piston-Connecting Rod Assembly B/RConn1 -- "CrodB-Crank Revolute Joint "/LConn1
  Piston B/RConn1 -- Piston-Connecting Rod Assembly B/LConn1
  Piston-Connecting Rod Assembly C/RConn1 -- "CrodC-Crank Revolute Joint "/LConn1
  Piston C/RConn1 -- Piston-Connecting Rod Assembly C/LConn1
  "CrodE-Crank Revolute Joint "/RConn1 -- Pentagonal Crank Plate/RConn3
  Piston D/RConn1 -- Piston-Connecting Rod Assembly D/LConn1
  Piston-Connecting Rod Assembly E/RConn1 -- "CrodE-Crank Revolute Joint "/LConn1
  Shaft/RConn1 -- Drive Shaft and Fly Wheel/LConn1
  "CrodB-Crank Revolute Joint "/RConn1 -- Pentagonal Crank Plate/LConn3

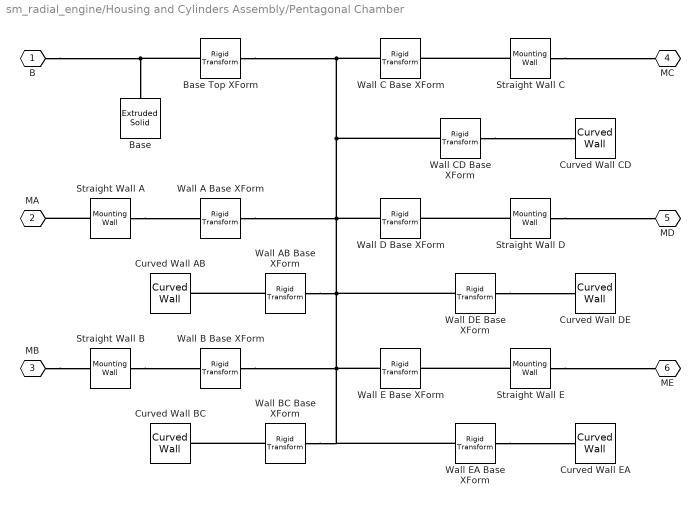
== system sm_radial_engine/Housing and Cylinders Assembly/Pentagonal Chamber ==
  Base : sm_lib/Body Elements/Extruded Solid  GraphicAmbientColor=[0.15 0.15 0.15 1.0]  BasedOnType=Density  CenterOfMass=[0 0 0]  CenterOfMassUnits=m  GraphicDiffuseColor=clr  ExportConvexHullGeometry=off  ExtrusionCrossSection=base_xsec  ExtrusionCrossSectionUnits=cm  Density=rho  DensityUnits=kg/(m^3)  DoExposeReferenceFrame=on  GraphicEmissiveColor=[0.0 0.0 0.0 1.0]  ExportEntireGeometry=off  ExtrusionLength=Tw  ExtrusionLengthUnits=cm  ExtrusionType=General  SerializedFrames=<Frames/>  MarkerShape=Sphere  MarkerSize=10  GraphicType=FromGeometry  InertiaType=CalculateFromGeometry  Mass=1  MassUnits=kg  MomentsOfInertia=[1 1 1]  MomentsOfInertiaUnits=kg*m^2  PolygonNumSides=3  GraphicOpacity=1.0  PolygonOuterRadius=1  PolygonOuterRadiusUnits=m  ProductsOfInertia=[0 0 0]  ProductsOfInertiaUnits=kg*m^2  GraphicShininess=75  GraphicSpecularColor=[0.5 0.5 0.5 1.0]  GraphicVisPropType=SimpleVisualProperties
  Base Top XForm : sm_lib/Frames and Transforms/Rigid Transform  TranslationMethod=StandardAxis  TranslationStandardOffset=Tw/2  TranslationLengthUnit=cm  TranslationStandardAxis=+Z  TranslationCartesianOffset=[0 0 0]  TranslationROffset=0  TranslationROffsetUnits=cm  TranslationZOffset=0  TranslationZOffsetUnits=cm  TranslationThetaOffset=36  TranslationThetaOffsetUnits=deg  RotationMethod=None  RotationAngleUnits=deg  RotationStandardAxis=+Z  RotationAngle=36  RotationArbitraryAxis=[0 0 1]  FollAlignAxisA=+Z  BaseAlignAxisA=+Y  FollAlignAxisB=+Y  BaseAlignAxisB=-X  RotationSequenceAxes=FollowerAxes  RotationSequence=XYX  RotationSequenceAngles=[0 0 0]  RotationSequenceAnglesUnits=deg  RotationMatrix=[1 0 0; 0 1 0; 0 0 1]
  Curved Wall AB : sm_radial_engine_lib/Curved Wall  Rw=Rcw  Tw=Tw  Hw=Hw  Aw=72  clr=clr  rho=rho
      settings: SourceProductBaseCode=MS
  Curved Wall BC : sm_radial_engine_lib/Curved Wall  Rw=Rcw  Tw=Tw  Hw=Hw  Aw=72  clr=clr  rho=rho
      settings: SourceProductBaseCode=MS
  Curved Wall CD : sm_radial_engine_lib/Curved Wall  Rw=Rcw  Tw=Tw  Hw=Hw  Aw=72  clr=clr  rho=rho
      settings: SourceProductBaseCode=MS
  Curved Wall DE : sm_radial_engine_lib/Curved Wall  Rw=Rcw  Tw=Tw  Hw=Hw  Aw=72  clr=clr  rho=rho
      settings: SourceProductBaseCode=MS
  Curved Wall EA : sm_radial_engine_lib/Curved Wall  Rw=Rcw  Tw=Tw  Hw=Hw  Aw=72  clr=clr  rho=rho
      settings: SourceProductBaseCode=MS
  Straight Wall A : sm_radial_engine_lib/Mounting Wall  Lw=Lw  Tw=Tw  Hw=Hw  Rm=Rm  clr=clr  rho=rho
      settings: SourceProductBaseCode=MS
  Straight Wall B : sm_radial_engine_lib/Mounting Wall  Lw=Lw  Tw=Tw  Hw=Hw  Rm=Rm  clr=clr  rho=rho
      settings: SourceProductBaseCode=MS
  Straight Wall C : sm_radial_engine_lib/Mounting Wall  Lw=Lw  Tw=Tw  Hw=Hw  Rm=Rm  clr=clr  rho=rho
      settings: SourceProductBaseCode=MS
  Straight Wall D : sm_radial_engine_lib/Mounting Wall  Lw=Lw  Tw=Tw  Hw=Hw  Rm=Rm  clr=clr  rho=rho
      settings: SourceProductBaseCode=MS
  Straight Wall E : sm_radial_engine_lib/Mounting Wall  Lw=Lw  Tw=Tw  Hw=Hw  Rm=Rm  clr=clr  rho=rho
      settings: SourceProductBaseCode=MS
  Wall A Base XForm : sm_lib/Frames and Transforms/Rigid Transform  TranslationMethod=Cylindrical  TranslationStandardOffset=25  TranslationLengthUnit=cm  TranslationStandardAxis=+Z  TranslationCartesianOffset=[0 0 0]  TranslationROffset=Rc  TranslationROffsetUnits=cm  TranslationZOffset=0  TranslationZOffsetUnits=cm  TranslationThetaOffset=0  TranslationThetaOffsetUnits=deg  RotationMethod=None  RotationAngleUnits=deg  RotationStandardAxis=+Z  RotationAngle=0  RotationArbitraryAxis=[0 0 1]  FollAlignAxisA=+Z  BaseAlignAxisA=+Y  FollAlignAxisB=+Y  BaseAlignAxisB=-X  RotationSequenceAxes=FollowerAxes  RotationSequence=XYX  RotationSequenceAngles=[0 0 0]  RotationSequenceAnglesUnits=deg  RotationMatrix=[1 0 0; 0 1 0; 0 0 1]
  Wall AB Base XForm : sm_lib/Frames and Transforms/Rigid Transform  TranslationMethod=Cylindrical  TranslationStandardOffset=25  TranslationLengthUnit=cm  TranslationStandardAxis=+Z  TranslationCartesianOffset=[0 0 0]  TranslationROffset=Dcw  TranslationROffsetUnits=cm  TranslationZOffset=0  TranslationZOffsetUnits=cm  TranslationThetaOffset=36  TranslationThetaOffsetUnits=deg  RotationMethod=StandardAxis  RotationAngleUnits=deg  RotationStandardAxis=+Z  RotationAngle=36  RotationArbitraryAxis=[0 0 1]  FollAlignAxisA=+Z  BaseAlignAxisA=+Y  FollAlignAxisB=+Y  BaseAlignAxisB=-X  RotationSequenceAxes=FollowerAxes  RotationSequence=XYX  RotationSequenceAngles=[0 0 0]  RotationSequenceAnglesUnits=deg  RotationMatrix=[1 0 0; 0 1 0; 0 0 1]
  Wall B Base XForm : sm_lib/Frames and Transforms/Rigid Transform  TranslationMethod=Cylindrical  TranslationStandardOffset=25  TranslationLengthUnit=cm  TranslationStandardAxis=+Z  TranslationCartesianOffset=[0 0 0]  TranslationROffset=Rc  TranslationROffsetUnits=cm  TranslationZOffset=0  TranslationZOffsetUnits=cm  TranslationThetaOffset=72  TranslationThetaOffsetUnits=deg  RotationMethod=StandardAxis  RotationAngleUnits=deg  RotationStandardAxis=+Z  RotationAngle=72  RotationArbitraryAxis=[0 0 1]  FollAlignAxisA=+Z  BaseAlignAxisA=+Y  FollAlignAxisB=+Y  BaseAlignAxisB=-X  RotationSequenceAxes=FollowerAxes  RotationSequence=XYX  RotationSequenceAngles=[0 0 0]  RotationSequenceAnglesUnits=deg  RotationMatrix=[1 0 0; 0 1 0; 0 0 1]
  Wall BC Base XForm : sm_lib/Frames and Transforms/Rigid Transform  TranslationMethod=Cylindrical  TranslationStandardOffset=25  TranslationLengthUnit=cm  TranslationStandardAxis=+Z  TranslationCartesianOffset=[0 0 0]  TranslationROffset=Dcw  TranslationROffsetUnits=cm  TranslationZOffset=0  TranslationZOffsetUnits=cm  TranslationThetaOffset=36+72  TranslationThetaOffsetUnits=deg  RotationMethod=StandardAxis  RotationAngleUnits=deg  RotationStandardAxis=+Z  RotationAngle=36+72  RotationArbitraryAxis=[0 0 1]  FollAlignAxisA=+Z  BaseAlignAxisA=+Y  FollAlignAxisB=+Y  BaseAlignAxisB=-X  RotationSequenceAxes=FollowerAxes  RotationSequence=XYX  RotationSequenceAngles=[0 0 0]  RotationSequenceAnglesUnits=deg  RotationMatrix=[1 0 0; 0 1 0; 0 0 1]
  Wall C Base XForm : sm_lib/Frames and Transforms/Rigid Transform  TranslationMethod=Cylindrical  TranslationStandardOffset=25  TranslationLengthUnit=cm  TranslationStandardAxis=+Z  TranslationCartesianOffset=[0 0 0]  TranslationROffset=Rc  TranslationROffsetUnits=cm  TranslationZOffset=0  TranslationZOffsetUnits=cm  TranslationThetaOffset=2*72  TranslationThetaOffsetUnits=deg  RotationMethod=StandardAxis  RotationAngleUnits=deg  RotationStandardAxis=+Z  RotationAngle=2*72  RotationArbitraryAxis=[0 0 1]  FollAlignAxisA=+Z  BaseAlignAxisA=+Y  FollAlignAxisB=+Y  BaseAlignAxisB=-X  RotationSequenceAxes=FollowerAxes  RotationSequence=XYX  RotationSequenceAngles=[0 0 0]  RotationSequenceAnglesUnits=deg  RotationMatrix=[1 0 0; 0 1 0; 0 0 1]
  Wall CD Base XForm : sm_lib/Frames and Transforms/Rigid Transform  TranslationMethod=Cylindrical  TranslationStandardOffset=25  TranslationLengthUnit=cm  TranslationStandardAxis=+Z  TranslationCartesianOffset=[0 0 0]  TranslationROffset=Dcw  TranslationROffsetUnits=cm  TranslationZOffset=0  TranslationZOffsetUnits=cm  TranslationThetaOffset=36+2*72  TranslationThetaOffsetUnits=deg  RotationMethod=StandardAxis  RotationAngleUnits=deg  RotationStandardAxis=+Z  RotationAngle=36+2*72  RotationArbitraryAxis=[0 0 1]  FollAlignAxisA=+Z  BaseAlignAxisA=+Y  FollAlignAxisB=+Y  BaseAlignAxisB=-X  RotationSequenceAxes=FollowerAxes  RotationSequence=XYX  RotationSequenceAngles=[0 0 0]  RotationSequenceAnglesUnits=deg  RotationMatrix=[1 0 0; 0 1 0; 0 0 1]
  Wall D Base XForm : sm_lib/Frames and Transforms/Rigid Transform  TranslationMethod=Cylindrical  TranslationStandardOffset=25  TranslationLengthUnit=cm  TranslationStandardAxis=+Z  TranslationCartesianOffset=[0 0 0]  TranslationROffset=Rc  TranslationROffsetUnits=cm  TranslationZOffset=0  TranslationZOffsetUnits=cm  TranslationThetaOffset=3*72  TranslationThetaOffsetUnits=deg  RotationMethod=StandardAxis  RotationAngleUnits=deg  RotationStandardAxis=+Z  RotationAngle=3*72  RotationArbitraryAxis=[0 0 1]  FollAlignAxisA=+Z  BaseAlignAxisA=+Y  FollAlignAxisB=+Y  BaseAlignAxisB=-X  RotationSequenceAxes=FollowerAxes  RotationSequence=XYX  RotationSequenceAngles=[0 0 0]  RotationSequenceAnglesUnits=deg  RotationMatrix=[1 0 0; 0 1 0; 0 0 1]
  Wall DE Base XForm : sm_lib/Frames and Transforms/Rigid Transform  TranslationMethod=Cylindrical  TranslationStandardOffset=25  TranslationLengthUnit=cm  TranslationStandardAxis=+Z  TranslationCartesianOffset=[0 0 0]  TranslationROffset=Dcw  TranslationROffsetUnits=cm  TranslationZOffset=0  TranslationZOffsetUnits=cm  TranslationThetaOffset=36+3*72  TranslationThetaOffsetUnits=deg  RotationMethod=StandardAxis  RotationAngleUnits=deg  RotationStandardAxis=+Z  RotationAngle=36+3*72  RotationArbitraryAxis=[0 0 1]  FollAlignAxisA=+Z  BaseAlignAxisA=+Y  FollAlignAxisB=+Y  BaseAlignAxisB=-X  RotationSequenceAxes=FollowerAxes  RotationSequence=XYX  RotationSequenceAngles=[0 0 0]  RotationSequenceAnglesUnits=deg  RotationMatrix=[1 0 0; 0 1 0; 0 0 1]
  Wall E Base XForm : sm_lib/Frames and Transforms/Rigid Transform  TranslationMethod=Cylindrical  TranslationStandardOffset=25  TranslationLengthUnit=cm  TranslationStandardAxis=+Z  TranslationCartesianOffset=[0 0 0]  TranslationROffset=Rc  TranslationROffsetUnits=cm  TranslationZOffset=0  TranslationZOffsetUnits=cm  TranslationThetaOffset=4*72  TranslationThetaOffsetUnits=deg  RotationMethod=StandardAxis  RotationAngleUnits=deg  RotationStandardAxis=+Z  RotationAngle=4*72  RotationArbitraryAxis=[0 0 1]  FollAlignAxisA=+Z  BaseAlignAxisA=+Y  FollAlignAxisB=+Y  BaseAlignAxisB=-X  RotationSequenceAxes=FollowerAxes  RotationSequence=XYX  RotationSequenceAngles=[0 0 0]  RotationSequenceAnglesUnits=deg  RotationMatrix=[1 0 0; 0 1 0; 0 0 1]
  Wall EA Base XForm : sm_lib/Frames and Transforms/Rigid Transform  TranslationMethod=Cylindrical  TranslationStandardOffset=25  TranslationLengthUnit=cm  TranslationStandardAxis=+Z  TranslationCartesianOffset=[0 0 0]  TranslationROffset=Dcw  TranslationROffsetUnits=cm  TranslationZOffset=0  TranslationZOffsetUnits=cm  TranslationThetaOffset=36+4*72  TranslationThetaOffsetUnits=deg  RotationMethod=StandardAxis  RotationAngleUnits=deg  RotationStandardAxis=+Z  RotationAngle=36+4*72  RotationArbitraryAxis=[0 0 1]  FollAlignAxisA=+Z  BaseAlignAxisA=+Y  FollAlignAxisB=+Y  BaseAlignAxisB=-X  RotationSequenceAxes=FollowerAxes  RotationSequence=XYX  RotationSequenceAngles=[0 0 0]  RotationSequenceAnglesUnits=deg  RotationMatrix=[1 0 0; 0 1 0; 0 0 1]
  B : PMIOPort  Side=Left
  MA : PMIOPort  Port=2  Side=Left
  MB : PMIOPort  Port=3  Side=Left
  MC : PMIOPort  Port=4  Side=Right
  MD : PMIOPort  Port=5  Side=Right
  ME : PMIOPort  Port=6  Side=Right
  connections:
  Straight Wall A/RConn1 -- MA/RConn1
  Straight Wall A/LConn1 -- Wall A Base XForm/RConn1
  Straight Wall B/LConn1 -- Wall B Base XForm/RConn1
  MB/RConn1 -- Straight Wall B/RConn1
  Straight Wall C/RConn1 -- MC/RConn1
  Straight Wall C/LConn1 -- Wall C Base XForm/RConn1
  Straight Wall D/RConn1 -- MD/RConn1
  Straight Wall D/LConn1 -- Wall D Base XForm/RConn1
  Straight Wall E/LConn1 -- Wall E Base XForm/RConn1
  Straight Wall E/RConn1 -- ME/RConn1
  Wall AB Base XForm/RConn1 -- Curved Wall AB/LConn1
  Wall BC Base XForm/RConn1 -- Curved Wall BC/LConn1
  Wall CD Base XForm/RConn1 -- Curved Wall CD/LConn1
  Wall DE Base XForm/RConn1 -- Curved Wall DE/LConn1
  Wall EA Base XForm/RConn1 -- Curved Wall EA/LConn1
  Wall A Base XForm/LConn1 -- Base Top XForm/RConn1 -- Wall C Base XForm/LConn1 -- Wall CD Base XForm/LConn1 -- Wall AB Base XForm/LConn1 -- Wall BC Base XForm/LConn1 -- Wall EA Base XForm/LConn1 -- Wall B Base XForm/LConn1 -- Wall E Base XForm/LConn1 -- Wall DE Base XForm/LConn1 -- Wall D Base XForm/LConn1
  B/RConn1 -- Base Top XForm/LConn1 -- Base/RConn1
